simulink subsystem "Mode_Select"  (R2022a)
settings: Solver=VariableStepAuto  StartTime=0.0  StopTime=10.0  RelTol=1e-3
undefined symbols (not defined in the file or in its folder): Pacemaker_Mode
libraries: simulink x18
settings Model: Creator=ivanl  LastModifiedBy=ivanl

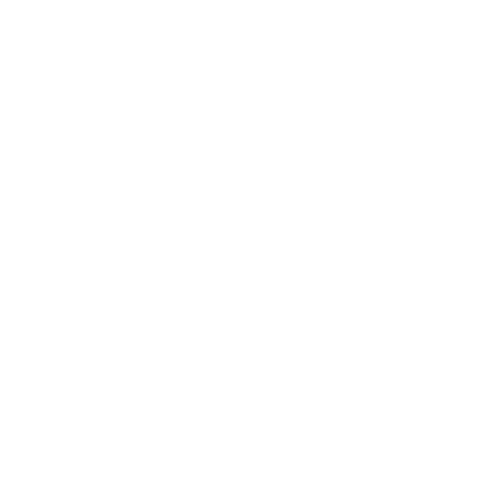
[thumbnail: Simulink's stored preview of the top-level diagram]
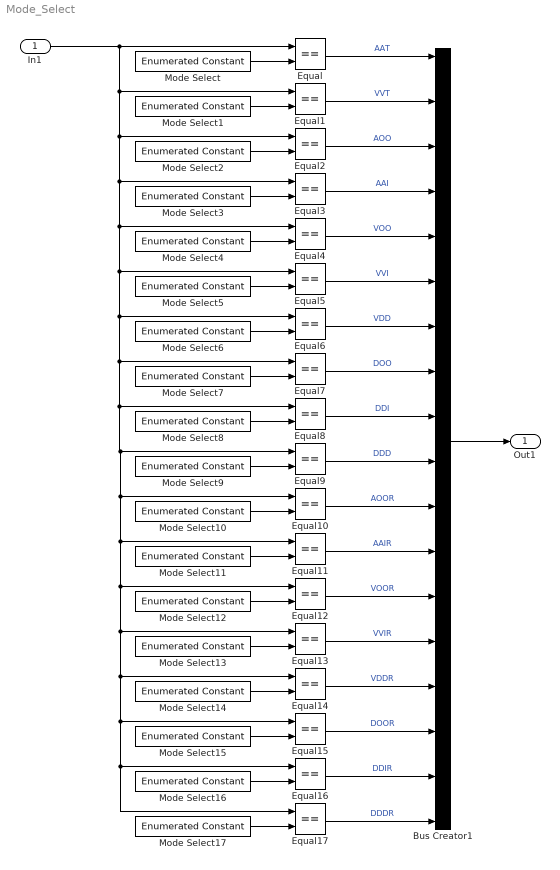
== system Mode_Select ==
  In1 : Inport
  Bus Creator1 : BusCreator  Inputs=18
  Equal{,1..17} (18 alike) : RelationalOperator  Operator===  OutDataTypeStr=boolean  RndMeth=Simplest  InputSameDT=off
  Mode Select : simulink/Sources/Enumerated Constant  OutDataTypeStr=Enum: Pacemaker_Mode  Value=Pacemaker_Mode.AAT  SampleTime=inf
  Mode Select1 : simulink/Sources/Enumerated Constant  OutDataTypeStr=Enum: Pacemaker_Mode  Value=Pacemaker_Mode.VVT  SampleTime=inf
  Mode Select10 : simulink/Sources/Enumerated Constant  OutDataTypeStr=Enum: Pacemaker_Mode  Value=Pacemaker_Mode.AOOR  SampleTime=inf
  Mode Select11 : simulink/Sources/Enumerated Constant  OutDataTypeStr=Enum: Pacemaker_Mode  Value=Pacemaker_Mode.AAIR  SampleTime=inf
  Mode Select12 : simulink/Sources/Enumerated Constant  OutDataTypeStr=Enum: Pacemaker_Mode  Value=Pacemaker_Mode.VOOR  SampleTime=inf
  Mode Select13 : simulink/Sources/Enumerated Constant  OutDataTypeStr=Enum: Pacemaker_Mode  Value=Pacemaker_Mode.VVIR  SampleTime=inf
  Mode Select14 : simulink/Sources/Enumerated Constant  OutDataTypeStr=Enum: Pacemaker_Mode  Value=Pacemaker_Mode.VDDR  SampleTime=inf
  Mode Select15 : simulink/Sources/Enumerated Constant  OutDataTypeStr=Enum: Pacemaker_Mode  Value=Pacemaker_Mode.DOOR  SampleTime=inf
  Mode Select16 : simulink/Sources/Enumerated Constant  OutDataTypeStr=Enum: Pacemaker_Mode  Value=Pacemaker_Mode.DDIR  SampleTime=inf
  Mode Select17 : simulink/Sources/Enumerated Constant  OutDataTypeStr=Enum: Pacemaker_Mode  Value=Pacemaker_Mode.DDDR  SampleTime=inf
  Mode Select2 : simulink/Sources/Enumerated Constant  OutDataTypeStr=Enum: Pacemaker_Mode  Value=Pacemaker_Mode.AOO  SampleTime=inf
  Mode Select3 : simulink/Sources/Enumerated Constant  OutDataTypeStr=Enum: Pacemaker_Mode  Value=Pacemaker_Mode.AAI  SampleTime=inf
  Mode Select4 : simulink/Sources/Enumerated Constant  OutDataTypeStr=Enum: Pacemaker_Mode  Value=Pacemaker_Mode.VOO  SampleTime=inf
  Mode Select5 : simulink/Sources/Enumerated Constant  OutDataTypeStr=Enum: Pacemaker_Mode  Value=Pacemaker_Mode.VVI  SampleTime=inf
  Mode Select6 : simulink/Sources/Enumerated Constant  OutDataTypeStr=Enum: Pacemaker_Mode  Value=Pacemaker_Mode.VDD  SampleTime=inf
  Mode Select7 : simulink/Sources/Enumerated Constant  OutDataTypeStr=Enum: Pacemaker_Mode  Value=Pacemaker_Mode.DOO  SampleTime=inf
  Mode Select8 : simulink/Sources/Enumerated Constant  OutDataTypeStr=Enum: Pacemaker_Mode  Value=Pacemaker_Mode.DDI  SampleTime=inf
  Mode Select9 : simulink/Sources/Enumerated Constant  OutDataTypeStr=Enum: Pacemaker_Mode  Value=Pacemaker_Mode.DDD  SampleTime=inf
  Out1 : Outport
  wires:
  Mode Select/1 -> Equal/2
  Mode Select1/1 -> Equal1/2
  Mode Select2/1 -> Equal2/2
  Mode Select3/1 -> Equal3/2
  Mode Select4/1 -> Equal4/2
  Mode Select5/1 -> Equal5/2
  Mode Select6/1 -> Equal6/2
  Mode Select8/1 -> Equal8/2
  Mode Select7/1 -> Equal7/2
  Mode Select9/1 -> Equal9/2
  Mode Select11/1 -> Equal11/2
  Mode Select10/1 -> Equal10/2
  Mode Select12/1 -> Equal12/2
  Mode Select14/1 -> Equal14/2
  Mode Select13/1 -> Equal13/2
  Mode Select15/1 -> Equal15/2
  Mode Select17/1 -> Equal17/2
  Mode Select16/1 -> Equal16/2
  In1/1 -> Equal/1, Equal1/1, Equal2/1, Equal3/1, Equal5/1, Equal6/1, Equal8/1, Equal9/1, Equal10/1, Equal11/1, Equal12/1, Equal13/1, Equal14/1, Equal15/1, Equal17/1, Equal16/1, Equal7/1, Equal4/1
  Equal4/1 -> Bus Creator1/5  "VOO"
  Equal3/1 -> Bus Creator1/4  "AAI"
  Equal2/1 -> Bus Creator1/3  "AOO"
  Equal1/1 -> Bus Creator1/2  "VVT"
  Equal/1 -> Bus Creator1/1  "AAT"
  Equal5/1 -> Bus Creator1/6  "VVI"
  Equal6/1 -> Bus Creator1/7  "VDD"
  Equal7/1 -> Bus Creator1/8  "DOO"
  Equal8/1 -> Bus Creator1/9  "DDI"
  Equal9/1 -> Bus Creator1/10  "DDD"
  Equal10/1 -> Bus Creator1/11  "AOOR"
  Equal11/1 -> Bus Creator1/12  "AAIR"
  Equal12/1 -> Bus Creator1/13  "VOOR"
  Equal13/1 -> Bus Creator1/14  "VVIR"
  Equal14/1 -> Bus Creator1/15  "VDDR"
  Equal15/1 -> Bus Creator1/16  "DOOR"
  Equal16/1 -> Bus Creator1/17  "DDIR"
  Equal17/1 -> Bus Creator1/18  "DDDR"
  Bus Creator1/1 -> Out1/1
